simulink model "lr_13_1"  (R2014b)
settings: Solver=ode45  StartTime=0.0  StopTime=30  RelTol=1e-3
libraries: simulink x1
settings Model: Creator=maksimka  LastModifiedBy=ADMIN

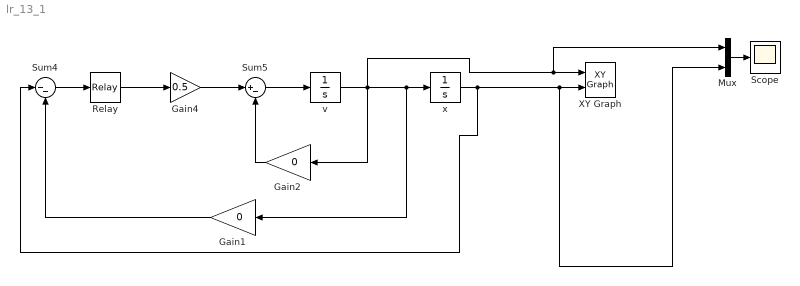
== system lr_13_1 ==
  Gain1 : Gain  Gain=0
  Gain2 : Gain  Gain=0
  Gain4 : Gain  Gain=0.5
  Mux : Mux  Inputs=2
  Relay : Relay  OnSwitchValue=0  OffSwitchValue=0  OffOutputValue=-1
  Scope : Scope
  Sum4 : Sum  Inputs=|--
  Sum5 : Sum  Inputs=|+-
  XY Graph : simulink/Sinks/XY Graph  xmin=-1  xmax=1  ymin=-1  ymax=1  st=-1
  v : Integrator
  x : Integrator  InitialCondition=5
  wires:
  Sum4/1 -> Relay/1
  Gain4/1 -> Sum5/1
  Sum5/1 -> v/1
  Relay/1 -> Gain4/1
  v/1 -> Mux/1, XY Graph/1, Gain2/1, Gain1/1, x/1
  Mux/1 -> Scope/1
  Gain1/1 -> Sum4/2
  Gain2/1 -> Sum5/2
  x/1 -> Sum4/1, Mux/2, XY Graph/2
